simulink model "task8_simulink"  (R2024b)
settings: Solver=ode45  StartTime=0.0  StopTime=100  RelTol=1e-6  AbsTol=1e-8
undefined symbols (not defined in the file): A, alpha_trim, B, C, D, h_trim, x_trim
settings Model: Creator=Admin  LastModifiedBy=david

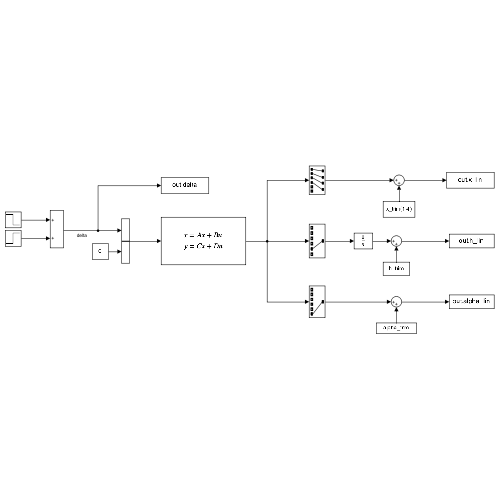
[thumbnail: Simulink's stored preview of the top-level diagram]
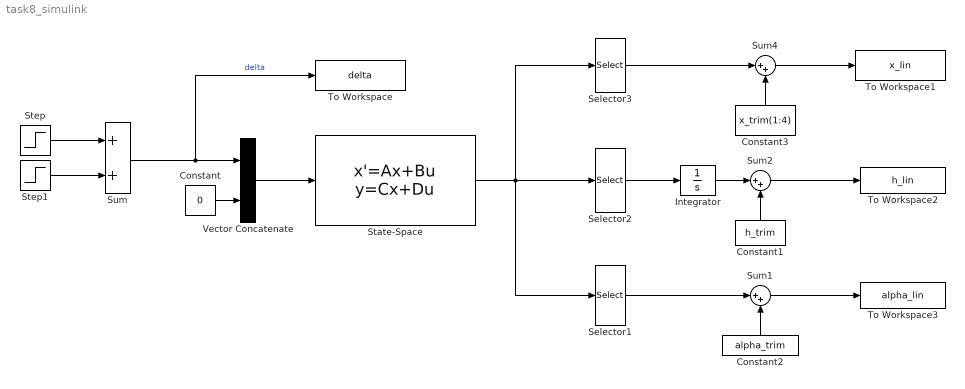
== system task8_simulink ==
  Constant : Constant  Value=0
  Constant1 : Constant  Value=h_trim
  Constant2 : Constant  Value=alpha_trim
  Constant3 : Constant  Value=x_trim(1:4)
  Integrator : Integrator
  Selector1 : Selector  InputPortWidth=6  IndexOptions=Index vector (dialog)  Indices=[6]  OutputSizes=1
  Selector2 : Selector  InputPortWidth=6  IndexOptions=Index vector (dialog)  Indices=[5]  OutputSizes=1
  Selector3 : Selector  InputPortWidth=6  IndexOptions=Index vector (dialog)  Indices=[1 2 3 4]  OutputSizes=1
  State-Space : StateSpace  A=A  B=B  C=C  D=D  InitialCondition=zeros(4,1)
  Step : Step  Time=5  After=- pi/180  SampleTime=0
  Step1 : Step  Time=10  After=(pi/180)  SampleTime=0
  Sum : Sum
  Sum1 : Sum  Inputs=|++
  Sum2 : Sum  Inputs=|++
  Sum4 : Sum  Inputs=|++
  To Workspace : ToWorkspace  VariableName=delta  SampleTime=-1
  To Workspace1 : ToWorkspace  VariableName=x_lin  SaveFormat=Structure  SampleTime=-1
      settings: Save2DSignal=2-D array (concatenate along first dimension)
  To Workspace2 : ToWorkspace  VariableName=h_lin  SampleTime=-1
      settings: Save2DSignal=2-D array (concatenate along first dimension)
  To Workspace3 : ToWorkspace  VariableName=alpha_lin  SampleTime=-1
  Vector Concatenate : Concatenate
  wires:
  Step/1 -> Sum/1
  Step1/1 -> Sum/2
  Sum/1 -> Vector Concatenate/1, To Workspace/1  "delta"
  Vector Concatenate/1 -> State-Space/1
  Constant/1 -> Vector Concatenate/2
  Constant3/1 -> Sum4/2
  Sum4/1 -> To Workspace1/1
  Selector2/1 -> Integrator/1
  Integrator/1 -> Sum2/1
  Sum1/1 -> To Workspace3/1
  Constant2/1 -> Sum1/2
  Selector1/1 -> Sum1/1
  Selector3/1 -> Sum4/1
  Sum2/1 -> To Workspace2/1
  Constant1/1 -> Sum2/2
  State-Space/1 -> Selector1/1, Selector2/1, Selector3/1
